simulink library "eml_lib"  (Simulink 6.0)
settings: Solver=ode45  SolverMode=SingleTasking  StartTime=0.0  StopTime=10.0  RelTol=1e-3
settings Model: Creator=The MathWorks Inc.  LastModifiedBy=batserve  ExtModeAutoUpdateStatusClock=off
settings DataIOCC: SignalLoggingName=logsOut
settings OptimizationCC: BooleanDataType=off
settings DebuggingCC: CheckExecutionContextPreStartOutputMsg=on  CheckExecutionContextRuntimeOutputMsg=on  SolverPrmCheckMsg=none
settings HardwareCC: TargetUnknown=on
settings ModelReferenceCC: UpdateModelReferenceTargets=IfOutOfDate

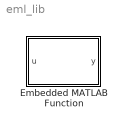
== system eml_lib ==
  Embedded MATLAB Function : Stateflow chart  PropExecContextAcrossSSBoundary=on

== matlab function Embedded MATLAB Function ==
  data: u input inherited; y output inherited
function y = fcn(u)
% This block supports an embeddable subset of the MATLAB language.
% See the help menu for details. 

y = u;
